simulink model "pv_guide"  (R2025b)
settings: Solver=VariableStepAuto  StartTime=0.0  StopTime=10.0  RelTol=1e-3

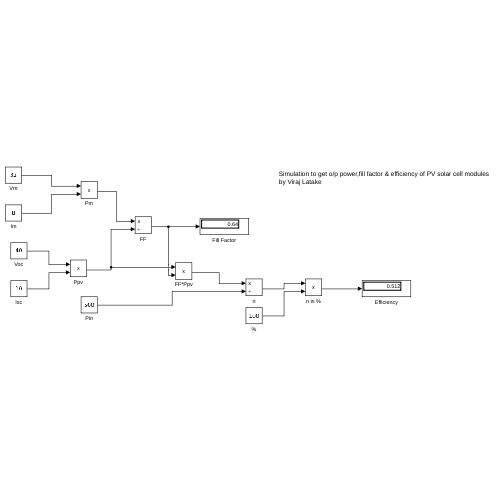
[thumbnail: Simulink's stored preview of the top-level diagram]
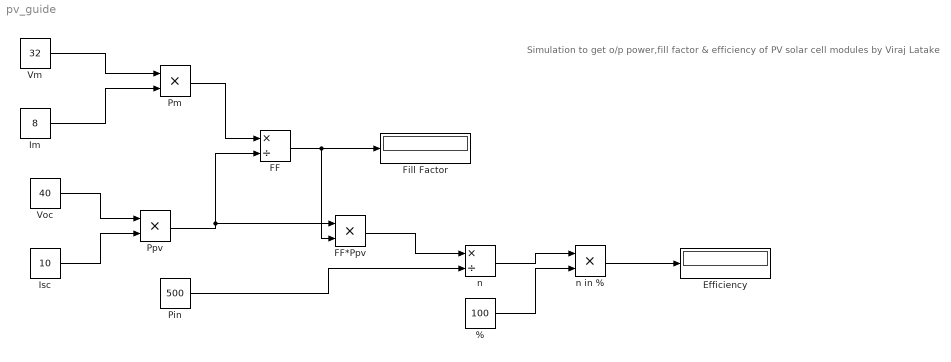
== system pv_guide ==
  note: Simulation to get o/p power,fill factor & efficiency of PV solar cell modules by Viraj Latake
  % : Constant  Value=100
  Efficiency : Display
  FF : Product  Inputs=*/
  FF*Ppv : Product
  Fill Factor : Display
  Im : Constant  Value=8
  Isc : Constant  Value=10
  Pin : Constant  Value=500
  Pm : Product
  Ppv : Product
  Vm : Constant  Value=32
  Voc : Constant  Value=40
  n : Product  Inputs=*/
  n in % : Product
  wires:
  Vm/1 -> Pm/1
  Im/1 -> Pm/2
  Voc/1 -> Ppv/1
  Isc/1 -> Ppv/2
  Pm/1 -> FF/1
  Ppv/1 -> FF/2, FF*Ppv/1
  FF/1 -> FF*Ppv/2, Fill Factor/1
  FF*Ppv/1 -> n/1
  Pin/1 -> n/2
  n/1 -> n in %/1
  %/1 -> n in %/2
  n in %/1 -> Efficiency/1
